simulink model "sampleModel351"  (R2021b)
settings: Solver=VariableStepAuto  StartTime=0.0  StopTime=10.0  RelTol=1e-3
undefined symbols (not defined in the file or in its folder): Newton, Raphson
libraries: simulink x8
settings Model: Creator=user  LastModifiedBy=user

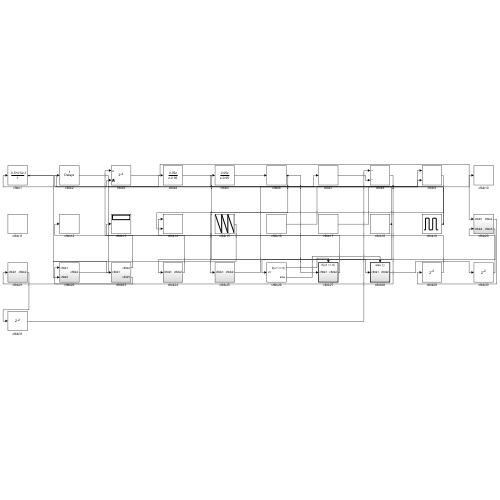
[thumbnail: Simulink's stored preview of the top-level diagram]
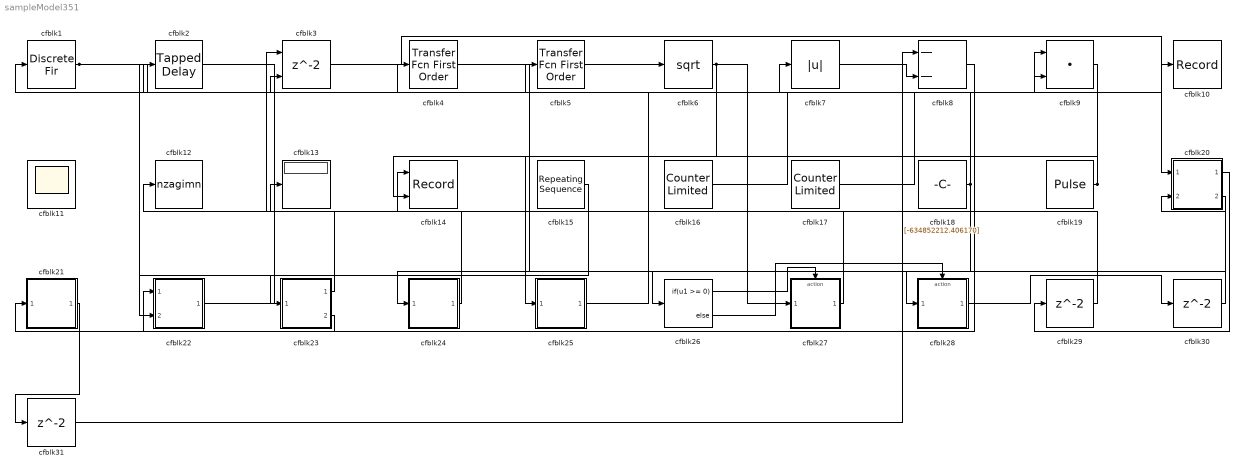
== system sampleModel351 ==
  cfblk1 : DiscreteFir  SampleTime=1
  cfblk10 : Record  FileSettingsInternal="{\"entries\":[{\"content\":{\"excelSettings\":{\"content\":{},\"type\":\"Streamout.ExcelSettings\"}},\"type\":\"Streamout.FileSettingStorage\",\"uuid\":\"fa105acb-6138-44d1-ba7d-028d937235ad\"}],\"packageUris\":[\"http://schema.mathworks.com/mf0/streamout_blocks/R2020a\"],\"version\":\"1.0\"}"  SignalsInternal="{\"entries\":[{\"content\":{\"signals\":[{\"content\":{\"blockPath\":[\"sampleModel351/cfblk10\"],\"channel\":[],\"dimensions\":[1],\"domain\":\"sampleModel351/cfblk10\",\"lineColor\":\"#a2142f\",\"plots\":[1],\"port\":1,\"sid\":[\"\"],\"signalID\":14629,\"signalName\":\"cfblk16\"},\"type\":\"RecordBlkView.Signal\",\"uuid\":\"18e12f01-e778-44ba-a0d1-b1385e119fc6\"}]},\"type\":\"RecordBlkView.InputSignals\",\"uuid\":\"daa177e1-477d-414b-8e15-bdb526d494a7\"}],\"packageUris\":[\"http://schema.mathworks.com/mf0/streamout_blocks/R2020a\"],\"version\":\"1.0\"}"  VisualizationBindings="{\"sparklinesplugin\":{\"info\":[{\"bindingParametersList\":[],\"subplotID\":1}]}}"
  cfblk11 : Scope
      settings: Floating=on
  cfblk12 : ToWorkspace  VariableName=nzagimn  SaveFormat=Timeseries  SampleTime=-1
  cfblk13 : Display
  cfblk14 : Record  FileSettingsInternal="{\"entries\":[{\"content\":{\"excelSettings\":{\"content\":{},\"type\":\"Streamout.ExcelSettings\"}},\"type\":\"Streamout.FileSettingStorage\",\"uuid\":\"e1215bf4-f163-4881-9128-e7d88cab1070\"}],\"packageUris\":[\"http://schema.mathworks.com/mf0/streamout_blocks/R2020a\"],\"version\":\"1.0\"}"  Layout=[1 1]  SignalsInternal="{\"entries\":[{\"content\":{\"signals\":[{\"content\":{\"blockPath\":[\"sampleModel351/cfblk14\"],\"channel\":[],\"dimensions\":[1],\"domain\":\"sampleModel351/cfblk14\",\"lineColor\":\"#a2142f\",\"plots\":[1],\"port\":1,\"sid\":[\"\"],\"signalID\":14621,\"signalName\":\"cfblk27\"},\"type\":\"RecordBlkView.Signal\",\"uuid\":\"bc6bf5eb-4561-4df8-9a91-f0c150a3e451\"},{\"content\":{\"blockPath\":[\"sampleModel351/cfblk14\"],\"channel\":[],\"dimensions\":[1],\"domain\":\"sampleModel351/cfblk14\",\"lineColor\":\"#139fff\",\"plots\":[1],\"port\":2,\"sid\":[\"\"],\"signalID\":14625,\"signalName\":\"cfblk9\"},\"type\":\"RecordBlkView.Signal\",\"uuid\":\"c060f1a2-c3d0-4e55-8568-84a09460571c\"}]},\"type\":\"RecordBlkView.InputSignals\",\"uuid\":\"3aa58f19-2ad2-410b-b46b-f2361a2e64fa\"}],\"packageUris\":[\"http://schema.mathworks.com/mf0/streamout_blocks/R2020a\"],\"version\":\"1.0\"}"  VisualizationBindings="{\"xyplotplugin\":{\"info\":[{\"series\":[{\"bindingParametersList\":[{\"parameter\":\"X-Axis\",\"signalID\":14621,\"signalName\":\"cfblk27\"},{\"parameter\":\"Y-Axis\",\"signalID\":14625,\"signalName\":\"cfblk9\"}],\"seriesID\":45997}],\"subplotID\":1}]}}"  CompatibilityTag=XY
  cfblk15 : simulink/Sources/Repeating Sequence  rep_seq_t=[0 2]  rep_seq_y=[797925960.282628, -826565874.384539]
  cfblk16 : simulink/Sources/Counter Limited  uplimit=[540.000000]  tsamp=-1
  cfblk17 : simulink/Sources/Counter Limited  uplimit=[508.000000]  tsamp=-1
  cfblk18 : Constant  Value=[-634852212.406170]  SampleTime=1
  cfblk19 : DiscretePulseGenerator  PulseType=Time based  Amplitude=[-360242174.239536]  Period=[9521285.729649]  PulseWidth=5  PhaseDelay=[5.000000]
  cfblk2 : simulink/Discrete/Tapped Delay  vinit=0.0  samptime=-1  NumDelays=1  DelayOrder=Oldest  includeCurrent=off
  cfblk20 : Subsystem
  cfblk21 : Subsystem
  cfblk22 : Subsystem
  cfblk23 : Subsystem
  cfblk24 : Subsystem
  cfblk25 : Subsystem
  cfblk26 : If  IfExpression=u1 >= 0  SampleTime=1
  cfblk27 : Subsystem  TreatAsAtomicUnit=on
  cfblk28 : Subsystem  TreatAsAtomicUnit=on
  cfblk29 : Delay  SampleTime=1
  cfblk3 : Delay  ShowEnablePort=on  SampleTime=1
      settings: InputPortMap=u0,e6
  cfblk30 : Delay  SampleTime=1
  cfblk31 : Delay  SampleTime=1
  cfblk4 : simulink/Discrete/Transfer Fcn First Order  PoleZ=0.95  ICPrevOutput=0.0  DoSatur=off
  cfblk5 : simulink/Discrete/Transfer Fcn First Order  PoleZ=0.95  ICPrevOutput=0.0  DoSatur=off
  cfblk6 : Sqrt  SaturateOnIntegerOverflow=on
  cfblk7 : Abs
  cfblk8 : Sum  Inputs=--
  cfblk9 : DotProduct  InputSameDT=on  OutDataTypeStr=Inherit: Inherit via internal rule
  wires:
  cfblk4/1 -> cfblk28/1(cfblk1)
  cfblk6/1 -> cfblk25/1(cfblk1), cfblk27/1(cfblk1)
  cfblk3/1 -> cfblk20/1(cfblk1)
  cfblk8/1 -> cfblk21/1(cfblk1)
  cfblk16/1 -> cfblk10/1
  cfblk17/1 -> cfblk9/1
  cfblk22/1(cfblk2) -> cfblk7/1
  cfblk24/1(cfblk2) -> cfblk13/1
  cfblk19/1 -> cfblk1/1, cfblk2/1
  cfblk18/1 -> cfblk5/1, cfblk24/1(cfblk1)
  cfblk7/1 -> cfblk8/2
  cfblk20/2(cfblk5) -> cfblk26/1
  cfblk2/1 -> cfblk4/1
  cfblk5/1 -> cfblk6/1
  cfblk23/1(cfblk2) -> cfblk12/1
  cfblk27/1(cfblk2) -> cfblk14/1
  cfblk23/2(cfblk5) -> cfblk22/1(cfblk1)
  cfblk1/1 -> cfblk3/2, cfblk23/1(cfblk1)
  cfblk9/1 -> cfblk14/2
  cfblk25/1(cfblk2) -> cfblk9/2
  cfblk15/1 -> cfblk22/2(cfblk5)
  cfblk26/1 -> cfblk27/Action
  cfblk26/2 -> cfblk28/Action
  cfblk20/1(cfblk2) -> cfblk29/1
  cfblk29/1 -> cfblk3/1
  cfblk28/1(cfblk2) -> cfblk30/1
  cfblk30/1 -> cfblk20/2(cfblk4)
  cfblk21/1(cfblk2) -> cfblk31/1
  cfblk31/1 -> cfblk8/1

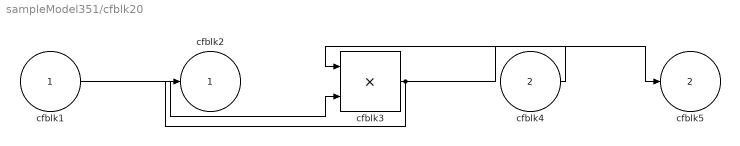
== system sampleModel351/cfblk20 ==
  cfblk1 : Inport
  cfblk4 : Inport  Port=2
  cfblk3 : Product  Inputs=**
  cfblk2 : Outport
  cfblk5 : Outport  Port=2
  wires:
  cfblk4/1 -> cfblk3/1
  cfblk1/1 -> cfblk3/2
  cfblk3/1 -> cfblk2/1, cfblk5/1

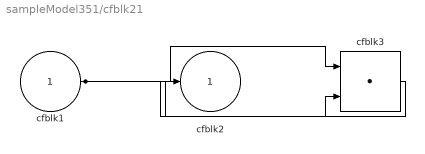
== system sampleModel351/cfblk21 ==
  cfblk1 : Inport
  cfblk3 : DotProduct  InputSameDT=on  OutDataTypeStr=Inherit: Inherit via internal rule
  cfblk2 : Outport
  wires:
  cfblk1/1 -> cfblk3/1, cfblk3/2
  cfblk3/1 -> cfblk2/1

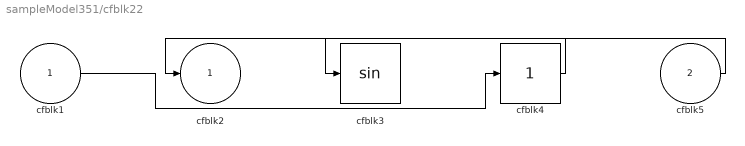
== system sampleModel351/cfblk22 ==
  cfblk1 : Inport
  cfblk5 : Inport  Port=2
  cfblk3 : Trigonometry
  cfblk4 : simulink/Math Operations/Slider Gain  gain=1  low=0  high=2
  cfblk2 : Outport
  wires:
  cfblk4/1 -> cfblk2/1
  cfblk1/1 -> cfblk4/1
  cfblk5/1 -> cfblk3/1

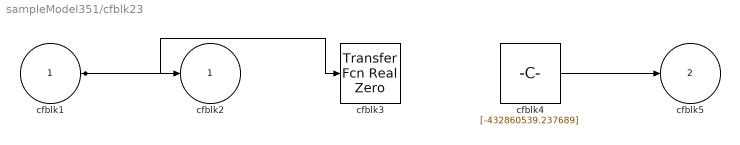
== system sampleModel351/cfblk23 ==
  cfblk1 : Inport
  cfblk3 : simulink/Discrete/Transfer Fcn Real Zero  ZeroZ=0.75  ICPrevInput=0.0  DoSatur=off
      settings: SourceProductBaseCode=SL
  cfblk4 : Constant  Value=[-432860539.237689]  SampleTime=1
  cfblk2 : Outport
  cfblk5 : Outport  Port=2
  wires:
  cfblk4/1 -> cfblk5/1
  cfblk1/1 -> cfblk2/1, cfblk3/1

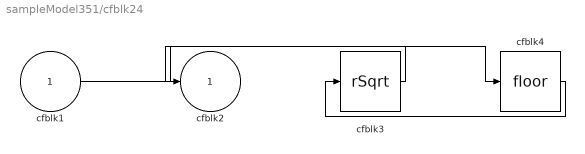
== system sampleModel351/cfblk24 ==
  cfblk1 : Inport
  cfblk3 : Sqrt  Operator=rSqrt  AlgorithmType=Newton-Raphson  SaturateOnIntegerOverflow=on
  cfblk4 : Rounding
  cfblk2 : Outport
  wires:
  cfblk1/1 -> cfblk4/1
  cfblk4/1 -> cfblk3/1
  cfblk3/1 -> cfblk2/1

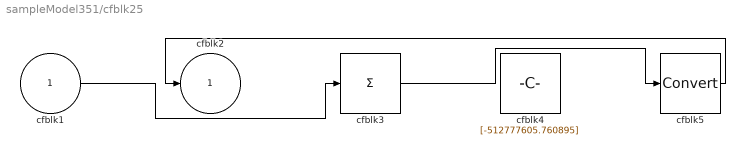
== system sampleModel351/cfblk25 ==
  cfblk1 : Inport
  cfblk3 : Sum  Inputs=+
  cfblk4 : Constant  Value=[-512777605.760895]  SampleTime=1
  cfblk5 : DataTypeConversion
  cfblk2 : Outport
  wires:
  cfblk1/1 -> cfblk3/1
  cfblk3/1 -> cfblk5/1
  cfblk5/1 -> cfblk2/1

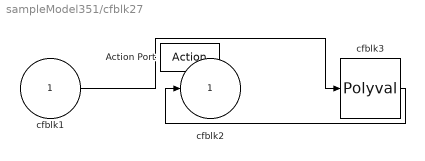
== system sampleModel351/cfblk27 ==
  cfblk1 : Inport
  Action Port : ActionPort  ActionPortLabel=if(u1 >= 0)
  cfblk3 : Polyval  Coefs=[ +2.081618890e-019, -1.441693666e-014, +4.719686976e-010, -8.536869453e-006, +1.621573104e-001, -8.087801117e+001 ]
  cfblk2 : Outport
  wires:
  cfblk3/1 -> cfblk2/1
  cfblk1/1 -> cfblk3/1

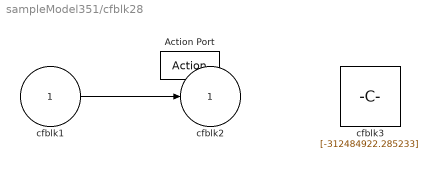
== system sampleModel351/cfblk28 ==
  cfblk1 : Inport
  Action Port : ActionPort  ActionPortLabel=else
  cfblk3 : Constant  Value=[-312484922.285233]  SampleTime=1
  cfblk2 : Outport
  wires:
  cfblk1/1 -> cfblk2/1
